simulink model "resistor_inductor_capacitor"  (R2024b)
settings: Solver=VariableStepAuto  StartTime=0.0  StopTime=10.0  RelTol=1e-3
values from neighbouring files (symbols this model uses):
  C = 100e-6    (= 0.0001)    [RLC_constants.m]
  R = 5    [RLC_constants.m]
settings Model: Creator=Aryan  LastModifiedBy=Aryan

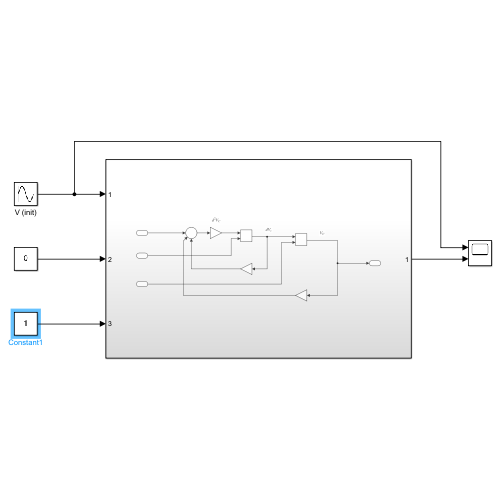
[thumbnail: Simulink's stored preview of the top-level diagram]
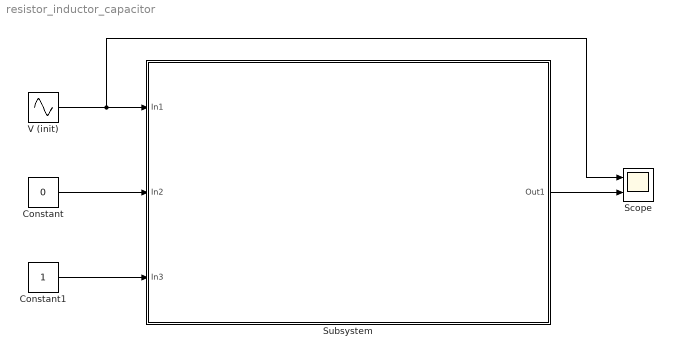
== system resistor_inductor_capacitor ==
  Constant : Constant  Value=0
  Constant1 : Constant
  Scope : Scope  NumInputPorts=2
  Subsystem : Subsystem
  V (init) : Sin  SampleTime=0
  wires:
  V (init)/1 -> Subsystem/1(In1), Scope/1
  Constant/1 -> Subsystem/2(In2)
  Constant1/1 -> Subsystem/3(In3)
  Subsystem/1(Out1) -> Scope/2

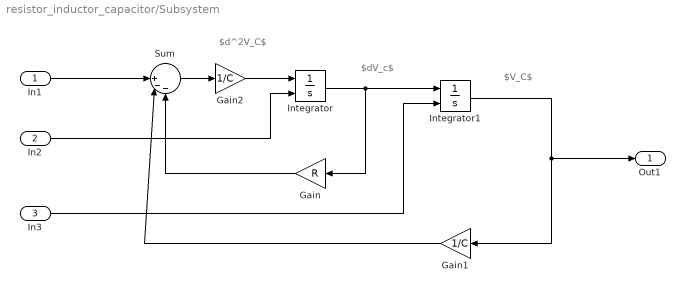
== system resistor_inductor_capacitor/Subsystem ==
  note: $V_C$
  note: $dV_c$
  note: $d^2V_C$
  In1 : Inport
  In2 : Inport  Port=2
  In3 : Inport  Port=3
  Gain : Gain  Gain=R
  Gain1 : Gain  Gain=1/C
  Gain2 : Gain  Gain=1/C
  Integrator : Integrator  InitialConditionSource=external
  Integrator1 : Integrator  InitialConditionSource=external
  Sum : Sum  Inputs=||+--
  Out1 : Outport
  wires:
  Integrator/1 -> Integrator1/1, Gain/1
  Integrator1/1 -> Out1/1, Gain1/1
  In3/1 -> Integrator1/2
  Gain2/1 -> Integrator/1
  Sum/1 -> Gain2/1
  Gain1/1 -> Sum/2
  Gain/1 -> Sum/3
  In2/1 -> Integrator/2
  In1/1 -> Sum/1
